simulink model "Traj_plt"  (R2023a)
settings: Solver=VariableStepAuto  StartTime=0.0  StopTime=inf  RelTol=1e-3
values from neighbouring files (symbols this model uses):
  beta = beta_i'.*task    [Compare1.m]    (also in Compare2.m; Final1.m; Final2.m; Final3.m)
undefined symbols (not defined in the file or in its folder): B_prev, Bst, Bst_prev, convertStringsToChars, dist_C, DroneMass, Earth, Gravity, h_ref, initialState, quad_pos, sinit, stack_size, task_mat, WGS84
libraries: slpidlib x66, aerolibconvert2 x11, aerolibtransform2 x11, uavalgslib x11, dspsrcs4 x1
(part 12 of 12)

== system Traj_plt/agent_9/Quad_1/Inner Loop and Plant Model/Low-FidelityModel/Position and Acceleration Control/Velocity Control1 ==
  Velocity Cmd : Inport
  QuadRotorState : Inport  Port=2
  Add1 : Sum  Inputs=+-
  Bus Selector1 : BusSelector  OutputSignals=WorldVelocity
  Data Type Conversion{,1..5} (6 alike) : DataTypeConversion  OutDataTypeStr=single  SaturateOnIntegerOverflow=off  RndMeth=Floor
  Demux1 : Demux  Outputs=3
  Mux : Mux  Inputs=3
  PID_Vx : slpidlib/PID Controller  Controller=PID  Form=Parallel  TimeDomain=Discrete-time  UseExternalTs=off  SampleTime=-1  IntegratorMethod=Forward Euler  FilterMethod=Forward Euler  ControllerParametersSource=internal  P=0.35  I=0  UseKiTs=off  D=0.1  N=10  UseFilter=on  TunerSelectOption=Transfer Function Based (PID Tuner App)  InitialConditionSource=internal  InitialConditionForIntegrator=0  InitialConditionForFilter=0  DifferentiatorICPrevScaledInput=0  ExternalReset=none  TrackingMode=off  Kt=1  LimitOutput=on  SatLimitsSource=internal  UpperSaturationLimit=1  LowerSaturationLimit=-1  LinearizeAsGain=on  AntiWindupMode=clamping  Kb=1  LimitIntegrator=off  UpperIntegratorSaturationLimit=inf  LowerIntegratorSaturationLimit=-inf  PGainOutDataTypeStr=single  PProdOutDataTypeStr=single  POutMin=[]  POutMax=[]  IGainOutDataTypeStr=single  IProdOutDataTypeStr=single  IOutMin=[]  IOutMax=[]  DGainOutDataTypeStr=single  DProdOutDataTypeStr=single  DOutMin=[]  DOutMax=[]  NGainOutDataTypeStr=single  NProdOutDataTypeStr=single  NOutMin=[]  NOutMax=[]  SumOutDataTypeStr=single  SumOutMin=[]  SumOutMax=[]  SaturationOutDataTypeStr=single  SaturationOutMin=[]  SaturationOutMax=[]  PParamMin=[]  PParamMax=[]  IParamMin=[]  IParamMax=[]  DParamMin=[]  DParamMax=[]  NParamMin=[]  NParamMax=[]  KbParamMin=[]  KbParamMax=[]  KtParamMin=[]  KtParamMax=[]  KbOutMin=[]  KbOutMax=[]  KtOutMin=[]  KtOutMax=[]  IntegratorOutMin=[]  IntegratorOutMax=[]  FilterOutMin=[]  FilterOutMax=[]  SumI1OutMin=SumI1OutMin  SumI1OutMax=SumI1OutMax  SumI2OutMin=[]  SumI2OutMax=[]  SumI3OutMin=[]  SumI3OutMax=[]  SumI4OutMin=[]  SumI4OutMax=[]  SumDOutMin=[]  SumDOutMax=[]  DifferentiatorOutMin=[]  DifferentiatorOutMax=[]  FilterDiffOutCoefMin=[]  FilterDiffOutCoefMax=[]  ReciprocalOutMin=[]  ReciprocalOutMax=[]  SumDenOutMin=[]  SumDenOutMax=[]  SumNumOutMin=[]  SumNumOutMax=[]  DivideOutMin=[]  DivideOutMax=[]  UdiffTsProdOutMin=[]  UdiffTsProdOutMax=[]  NTsProdOutMin=[]  NTsProdOutMax=[]  UintegralTsProdOutMin=[]  UintegralTsProdOutMax=[]  UngainTsProdOutMin=[]  UngainTsProdOutMax=[]  ClampingZeroOutDataTypeStr=Inherit: Inherit via back propagation  ClampingZeroOutMin=[]  ClampingZeroOutMax=[]  FilterDenConstantOutDataTypeStr=Inherit: Inherit via back propagation  FilterDenConstantOutMin=[]  FilterDenConstantOutMax=[]  PCopyOutDataTypeStr=Inherit: Inherit via back propagation  PCopyOutMin=[]  PCopyOutMax=[]  NCopyOutDataTypeStr=Inherit: Inherit via back propagation  NCopyOutMin=[]  NCopyOutMax=[]  IntegratorContinuousStateAttributes=''  IntegratorStateMustResolveToSignalObject=off  IntegratorRTWStateStorageClass=Auto  FilterContinuousStateAttributes=''  FilterStateMustResolveToSignalObject=off  FilterRTWStateStorageClass=Auto  ParallelPVariant=InternalParameters  IdealPVariant=Disabled  IVariant=InternalParameters  DVariant=InternalParameters  IntegratorVariant=Discrete  SatVariant=Enabled  AWVariant=DiscClampingParallel  PCopyVariant=Disabled  TRVariant=Disabled  FdbkBlocksVariant=Forward  IdealPFdbkVariant=Disabled  SatFdbkVariant=Disabled  DerivativeFilterVariant=ForwardEulerFilter  NVariant=InternalParameters  NCopyVariant=Disabled  FilterICVariant=InternalICsFilter  IntegratorICVariant=InternalICs  ExternalResetVariant=Disabled  TRSumVariant=Passthrough  SumFdbkVariant=Disabled  SumVariant=Sum_PID  TsampFilterVariant=InternalTs  TsampNgainVariant=Passthrough  TsampIntegralVariant=Disabled_SignalSpec  ExternalSaturationOutDataTypeStr=Inherit: Same as second input
      settings: AttributesFormatString=P: %<P>, I: %<I>, D:%<D>
  PID_Vy : slpidlib/PID Controller  Controller=PID  Form=Parallel  TimeDomain=Discrete-time  UseExternalTs=off  SampleTime=-1  IntegratorMethod=Forward Euler  FilterMethod=Forward Euler  ControllerParametersSource=internal  P=0.35  I=0  UseKiTs=off  D=0.1  N=10  UseFilter=on  TunerSelectOption=Transfer Function Based (PID Tuner App)  InitialConditionSource=internal  InitialConditionForIntegrator=0  InitialConditionForFilter=0  DifferentiatorICPrevScaledInput=0  ExternalReset=none  TrackingMode=off  Kt=1  LimitOutput=on  SatLimitsSource=internal  UpperSaturationLimit=1  LowerSaturationLimit=-1  LinearizeAsGain=on  AntiWindupMode=clamping  Kb=1  LimitIntegrator=off  UpperIntegratorSaturationLimit=inf  LowerIntegratorSaturationLimit=-inf  POutMin=[]  POutMax=[]  IOutMin=[]  IOutMax=[]  DOutMin=[]  DOutMax=[]  NOutMin=[]  NOutMax=[]  SumOutMin=[]  SumOutMax=[]  SaturationOutMin=[]  SaturationOutMax=[]  PParamMin=[]  PParamMax=[]  IParamMin=[]  IParamMax=[]  DParamMin=[]  DParamMax=[]  NParamMin=[]  NParamMax=[]  KbParamMin=[]  KbParamMax=[]  KtParamMin=[]  KtParamMax=[]  KbOutMin=[]  KbOutMax=[]  KtOutMin=[]  KtOutMax=[]  IntegratorOutMin=[]  IntegratorOutMax=[]  FilterOutMin=[]  FilterOutMax=[]  SumI1OutMin=SumI1OutMin  SumI1OutMax=SumI1OutMax  SumI2OutMin=[]  SumI2OutMax=[]  SumI3OutMin=[]  SumI3OutMax=[]  SumI4OutMin=[]  SumI4OutMax=[]  SumDOutMin=[]  SumDOutMax=[]  DifferentiatorOutMin=[]  DifferentiatorOutMax=[]  FilterDiffOutCoefMin=[]  FilterDiffOutCoefMax=[]  ReciprocalOutMin=[]  ReciprocalOutMax=[]  SumDenOutMin=[]  SumDenOutMax=[]  SumNumOutMin=[]  SumNumOutMax=[]  DivideOutMin=[]  DivideOutMax=[]  UdiffTsProdOutMin=[]  UdiffTsProdOutMax=[]  NTsProdOutMin=[]  NTsProdOutMax=[]  UintegralTsProdOutMin=[]  UintegralTsProdOutMax=[]  UngainTsProdOutMin=[]  UngainTsProdOutMax=[]  ClampingZeroOutDataTypeStr=Inherit: Inherit via back propagation  ClampingZeroOutMin=[]  ClampingZeroOutMax=[]  FilterDenConstantOutDataTypeStr=Inherit: Inherit via back propagation  FilterDenConstantOutMin=[]  FilterDenConstantOutMax=[]  PCopyOutDataTypeStr=Inherit: Inherit via back propagation  PCopyOutMin=[]  PCopyOutMax=[]  NCopyOutDataTypeStr=Inherit: Inherit via back propagation  NCopyOutMin=[]  NCopyOutMax=[]  IntegratorContinuousStateAttributes=''  IntegratorStateMustResolveToSignalObject=off  IntegratorRTWStateStorageClass=Auto  FilterContinuousStateAttributes=''  FilterStateMustResolveToSignalObject=off  FilterRTWStateStorageClass=Auto  ParallelPVariant=InternalParameters  IdealPVariant=Disabled  IVariant=InternalParameters  DVariant=InternalParameters  IntegratorVariant=Discrete  SatVariant=Enabled  AWVariant=DiscClampingParallel  PCopyVariant=Disabled  TRVariant=Disabled  FdbkBlocksVariant=Forward  IdealPFdbkVariant=Disabled  SatFdbkVariant=Disabled  DerivativeFilterVariant=ForwardEulerFilter  NVariant=InternalParameters  NCopyVariant=Disabled  FilterICVariant=InternalICsFilter  IntegratorICVariant=InternalICs  ExternalResetVariant=Disabled  TRSumVariant=Passthrough  SumFdbkVariant=Disabled  SumVariant=Sum_PID  TsampFilterVariant=InternalTs  TsampNgainVariant=Passthrough  TsampIntegralVariant=Disabled_SignalSpec  ExternalSaturationOutDataTypeStr=Inherit: Same as second input
      settings: AttributesFormatString=P: %<P>, I: %<I>, D:%<D>
  PID_Vz : slpidlib/PID Controller  Controller=PID  Form=Parallel  TimeDomain=Discrete-time  UseExternalTs=off  SampleTime=-1  IntegratorMethod=Forward Euler  FilterMethod=Forward Euler  ControllerParametersSource=internal  P=6.8  I=0  UseKiTs=off  D=2.5  N=14.495  UseFilter=on  TunerSelectOption=Transfer Function Based (PID Tuner App)  InitialConditionSource=internal  InitialConditionForIntegrator=0  InitialConditionForFilter=0  DifferentiatorICPrevScaledInput=0  ExternalReset=none  TrackingMode=off  Kt=1  LimitOutput=on  SatLimitsSource=internal  UpperSaturationLimit=2  LowerSaturationLimit=-2  LinearizeAsGain=on  AntiWindupMode=clamping  Kb=1  LimitIntegrator=off  UpperIntegratorSaturationLimit=inf  LowerIntegratorSaturationLimit=-inf  POutMin=[]  POutMax=[]  IOutMin=[]  IOutMax=[]  DOutMin=[]  DOutMax=[]  NOutMin=[]  NOutMax=[]  SumOutMin=[]  SumOutMax=[]  SaturationOutMin=[]  SaturationOutMax=[]  PParamMin=[]  PParamMax=[]  IParamMin=[]  IParamMax=[]  DParamMin=[]  DParamMax=[]  NParamMin=[]  NParamMax=[]  KbParamMin=[]  KbParamMax=[]  KtParamMin=[]  KtParamMax=[]  KbOutMin=[]  KbOutMax=[]  KtOutMin=[]  KtOutMax=[]  IntegratorOutMin=[]  IntegratorOutMax=[]  FilterOutMin=[]  FilterOutMax=[]  SumI1OutMin=SumI1OutMin  SumI1OutMax=SumI1OutMax  SumI2OutMin=[]  SumI2OutMax=[]  SumI3OutMin=[]  SumI3OutMax=[]  SumI4OutMin=[]  SumI4OutMax=[]  SumDOutMin=[]  SumDOutMax=[]  DifferentiatorOutMin=[]  DifferentiatorOutMax=[]  FilterDiffOutCoefMin=[]  FilterDiffOutCoefMax=[]  ReciprocalOutMin=[]  ReciprocalOutMax=[]  SumDenOutMin=[]  SumDenOutMax=[]  SumNumOutMin=[]  SumNumOutMax=[]  DivideOutMin=[]  DivideOutMax=[]  UdiffTsProdOutMin=[]  UdiffTsProdOutMax=[]  NTsProdOutMin=[]  NTsProdOutMax=[]  UintegralTsProdOutMin=[]  UintegralTsProdOutMax=[]  UngainTsProdOutMin=[]  UngainTsProdOutMax=[]  ClampingZeroOutDataTypeStr=Inherit: Inherit via back propagation  ClampingZeroOutMin=[]  ClampingZeroOutMax=[]  FilterDenConstantOutDataTypeStr=Inherit: Inherit via back propagation  FilterDenConstantOutMin=[]  FilterDenConstantOutMax=[]  PCopyOutDataTypeStr=Inherit: Inherit via back propagation  PCopyOutMin=[]  PCopyOutMax=[]  NCopyOutDataTypeStr=Inherit: Inherit via back propagation  NCopyOutMin=[]  NCopyOutMax=[]  IntegratorContinuousStateAttributes=''  IntegratorStateMustResolveToSignalObject=off  IntegratorRTWStateStorageClass=Auto  FilterContinuousStateAttributes=''  FilterStateMustResolveToSignalObject=off  FilterRTWStateStorageClass=Auto  ParallelPVariant=InternalParameters  IdealPVariant=Disabled  IVariant=InternalParameters  DVariant=InternalParameters  IntegratorVariant=Discrete  SatVariant=Enabled  AWVariant=DiscClampingParallel  PCopyVariant=Disabled  TRVariant=Disabled  FdbkBlocksVariant=Forward  IdealPFdbkVariant=Disabled  SatFdbkVariant=Disabled  DerivativeFilterVariant=ForwardEulerFilter  NVariant=InternalParameters  NCopyVariant=Disabled  FilterICVariant=InternalICsFilter  IntegratorICVariant=InternalICs  ExternalResetVariant=Disabled  TRSumVariant=Passthrough  SumFdbkVariant=Disabled  SumVariant=Sum_PID  TsampFilterVariant=InternalTs  TsampNgainVariant=Passthrough  TsampIntegralVariant=Disabled_SignalSpec  ExternalSaturationOutDataTypeStr=Inherit: Same as second input
      settings: AttributesFormatString=P: %<P>, I: %<I>, D:%<D>
  Accel Cmd : Outport
  wires:
  Add1/1 -> Demux1/1  "Velocity Error"
  PID_Vz/1 -> Data Type Conversion/1
  Demux1/1 -> Data Type Conversion4/1
  PID_Vy/1 -> Data Type Conversion1/1
  Velocity Cmd/1 -> Add1/1
  Demux1/3 -> Data Type Conversion5/1
  Mux/1 -> Accel Cmd/1
  PID_Vx/1 -> Data Type Conversion2/1
  Demux1/2 -> Data Type Conversion3/1
  Bus Selector1/1 -> Add1/2  "<WorldVelocity>"
  QuadRotorState/1 -> Bus Selector1/1
  Data Type Conversion/1 -> Mux/3
  Data Type Conversion1/1 -> Mux/2
  Data Type Conversion2/1 -> Mux/1
  Data Type Conversion3/1 -> PID_Vy/1
  Data Type Conversion4/1 -> PID_Vx/1
  Data Type Conversion5/1 -> PID_Vz/1

== matlab function Traj_plt/agent_11/Quad_1/Inner Loop and Plant Model/Low-FidelityModel/Assemble UAV State Bus/Generate GPS Data/Embedded MATLAB Function1 ==
  data: cog output; Vn input; Ve input
function cog = getCOG(Vn, Ve)
% This block supports an embeddable subset of the MATLAB language.
% See the help menu for details. 

cog = atan2(Ve,Vn);
if cog < 0;
    cog = cog + 2*pi;
end

== matlab function Traj_plt/MATLAB Function ==
  data: ag_no input; h output; d output; h_ref parameter; dist_C parameter
function [h,d] = fcn(ag_no, h_ref, dist_C)
h = h_ref(ag_no);
d = dist_C(ag_no);

== matlab function Traj_plt/agent_11/Quad_1/Inner Loop and Plant Model/Low-FidelityModel/Position and Acceleration Control/Attitude Control/Multirotor Acceleration Control ==
  data: acc input; roll output; pitch output; yaw input; Gravity parameter
function [roll, pitch] = accControl(acc, yaw, Gravity)

    xddot = acc(1);
    yddot = acc(2);
    zddot = acc(3);
    
    pitch = atan2((-xddot*cos(yaw)-yddot*sin(yaw)), ( -zddot + Gravity));
    roll = atan2(((-xddot*sin(yaw)+yddot*cos(yaw))*cos(pitch)), (-zddot+Gravity));
    
end

== matlab function Traj_plt/agent_11/Quad_1/Inner Loop and Plant Model/Low-FidelityModel/Position and Acceleration Control/Attitude Control/Multirotor Thrust Control ==
  data: acc input; pitch input; thrust output; roll input; DroneMass parameter; Gravity parameter
function thrust  = thrustControl(acc, pitch, roll, DroneMass, Gravity)

    zddot = acc(3);
    
    thrust = DroneMass*(-zddot+Gravity)/(cos(pitch)*cos(roll));
end

== matlab function Traj_plt/Fire_dyn ==
  data: srate output; beta input; s input
function srate = fcn(beta,s)
Fir_pts = [80,100;120,100]';
alpha = [1.2,1.5];
sinit = [2.1,1.2];
k = 0.6;
srate = k.*alpha.*sqrt(s)'-beta';
circle(Fir_pts(1,1),Fir_pts(2,1),sqrt(s(1)/pi),beta(1),s)
hold on
circle(Fir_pts(1,2),Fir_pts(2,2),sqrt(s(2)/pi),beta(2),s)
y=0;

== stateflow chart Traj_plt/Chart2 ==
  state Stat_assign
    Beta = Bst_prev*beta';
    %Bst = Bst_prev;
  state B_assign1
    Bst == task_mat(j,:,:);
  state B_assign
    Beta = Bst * beta';
  (default) -> Stat_assign
  Stat_assign -> B_assign : after(10,sec){j=1}
  B_assign -> B_assign1 : after(10,sec){j = j + 1}
  B_assign1 -> B_assign : after(1,sec)
  data: task_mat parameter; Bst_prev parameter; Bst parameter; Beta output; j output; beta parameter

== matlab function Traj_plt/agent_1/Quad_1/Inner Loop and Plant Model/Low-FidelityModel/Assemble UAV State Bus/Generate GPS Data/Embedded MATLAB Function1 ==
  data: cog output; Vn input; Ve input
function cog = getCOG(Vn, Ve)
% This block supports an embeddable subset of the MATLAB language.
% See the help menu for details. 

cog = atan2(Ve,Vn);
if cog < 0;
    cog = cog + 2*pi;
end

== matlab function Traj_plt/agent_1/Quad_1/Inner Loop and Plant Model/Low-FidelityModel/Position and Acceleration Control/Attitude Control/Multirotor Acceleration Control ==
  data: acc input; roll output; pitch output; yaw input; Gravity parameter
function [roll, pitch] = accControl(acc, yaw, Gravity)

    xddot = acc(1);
    yddot = acc(2);
    zddot = acc(3);
    
    pitch = atan2((-xddot*cos(yaw)-yddot*sin(yaw)), ( -zddot + Gravity));
    roll = atan2(((-xddot*sin(yaw)+yddot*cos(yaw))*cos(pitch)), (-zddot+Gravity));
    
end

== matlab function Traj_plt/agent_1/Quad_1/Inner Loop and Plant Model/Low-FidelityModel/Position and Acceleration Control/Attitude Control/Multirotor Thrust Control ==
  data: acc input; pitch input; thrust output; roll input; DroneMass parameter; Gravity parameter
function thrust  = thrustControl(acc, pitch, roll, DroneMass, Gravity)

    zddot = acc(3);
    
    thrust = DroneMass*(-zddot+Gravity)/(cos(pitch)*cos(roll));
end

== matlab function Traj_plt/MATLAB Function1 ==
  data: ag_no input; h output; d output; h_ref parameter; dist_C parameter
function [h,d] = fcn(ag_no, h_ref, dist_C)
h = h_ref(ag_no);
d = dist_C(ag_no);

== stateflow chart Traj_plt/agent_1/Chart2 ==
  state Stat_assign
    B = B_prev(ag_no);
  state B_assign1
    B = task_mat(j,ag_no,1);
  state B_assign
    B;
  (default) -> Stat_assign
  Stat_assign -> B_assign : after(10,sec){j=1}
  B_assign -> B_assign1 : after(10,sec){j = j + 1}
  B_assign1 -> B_assign : after(1,sec)
  data: B output; task_mat parameter; ag_no input; B_prev parameter; j output

== stateflow chart Traj_plt/agent_2/Chart1 ==
  state Fire_pt_1
    state set_1
      waypoint =[x-d,y-d,h; x+d,y-d,h;x+d,y+d,h;x-d,y+d,h];
    state set_2
      waypoint =[ x-d,y-d,h-0.1; x+d,y-d,h-0.1;x+d,y+d,h-0.1;x-d,y+d,h-0.1];
    Fire_pt_1.set_1 -> Fire_pt_1.set_2 : [meet==1]
    (default) -> Fire_pt_1.set_1
    Fire_pt_1.set_2 -> Fire_pt_1.set_1 : [meet==1]
  state Fire_pt_2
    state set_1
      waypoint =[a-d,b-d,g; a+d,b-d,g;a+d,b+d,g;a-d,b+d,g];
    state set_2
      waypoint = [ a-d,b-d,h-0.1; a+d,b-d,h-0.1;a+d,b+d,h-0.1;a-d,b+d,h-0.1];
    (default) -> Fire_pt_2.set_1
    Fire_pt_2.set_1 -> Fire_pt_2.set_2 : [meet==1]
    Fire_pt_2.set_2 -> Fire_pt_2.set_1 : [meet==1]
  (default) -> Fire_pt_1
  Fire_pt_1 -> Fire_pt_2 : [Assign==1]
  Fire_pt_2 -> Fire_pt_1 : [Assign==0]
  data: waypoint output; Assign input; a input; b input; g input; x input; h input; y input; d input; meet input

== stateflow chart Traj_plt/agent_2/Chart2 ==
  state Stat_assign
    B = B_prev(ag_no);
  state B_assign1
    B = task_mat(j,ag_no,1);
  state B_assign
    B;
  (default) -> Stat_assign
  Stat_assign -> B_assign : after(10,sec){j=1}
  B_assign -> B_assign1 : after(10,sec){j = j + 1}
  B_assign1 -> B_assign : after(1,sec)
  data: B output; task_mat parameter; ag_no input; B_prev parameter; j output

== matlab function Traj_plt/agent_2/MATLAB Function ==
  data: Assign output; B input
function Assign = fcn(B)
if (B==1)
    Assign=0;
else
    Assign=1;
end

== matlab function Traj_plt/agent_2/Quad_1/Inner Loop and Plant Model/Low-FidelityModel/Assemble UAV State Bus/Generate GPS Data/Embedded MATLAB Function1 ==
  data: cog output; Vn input; Ve input
function cog = getCOG(Vn, Ve)
% This block supports an embeddable subset of the MATLAB language.
% See the help menu for details. 

cog = atan2(Ve,Vn);
if cog < 0;
    cog = cog + 2*pi;
end

== matlab function Traj_plt/agent_2/Quad_1/Inner Loop and Plant Model/Low-FidelityModel/Position and Acceleration Control/Attitude Control/Multirotor Acceleration Control ==
  data: acc input; roll output; pitch output; yaw input; Gravity parameter
function [roll, pitch] = accControl(acc, yaw, Gravity)

    xddot = acc(1);
    yddot = acc(2);
    zddot = acc(3);
    
    pitch = atan2((-xddot*cos(yaw)-yddot*sin(yaw)), ( -zddot + Gravity));
    roll = atan2(((-xddot*sin(yaw)+yddot*cos(yaw))*cos(pitch)), (-zddot+Gravity));
    
end

== matlab function Traj_plt/agent_2/Quad_1/Inner Loop and Plant Model/Low-FidelityModel/Position and Acceleration Control/Attitude Control/Multirotor Thrust Control ==
  data: acc input; pitch input; thrust output; roll input; DroneMass parameter; Gravity parameter
function thrust  = thrustControl(acc, pitch, roll, DroneMass, Gravity)

    zddot = acc(3);
    
    thrust = DroneMass*(-zddot+Gravity)/(cos(pitch)*cos(roll));
end

== matlab function Traj_plt/MATLAB Function2 ==
  data: ag_no input; h output; d output; h_ref parameter; dist_C parameter
function [h,d] = fcn(ag_no, h_ref, dist_C)
h = h_ref(ag_no);
d = dist_C(ag_no);

== stateflow chart Traj_plt/agent_3/Chart1 ==
  state Fire_pt_1
    state set_1
      waypoint =[x-d,y-d,h; x+d,y-d,h;x+d,y+d,h;x-d,y+d,h];
    state set_2
      waypoint =[ x-d,y-d,h-0.1; x+d,y-d,h-0.1;x+d,y+d,h-0.1;x-d,y+d,h-0.1];
    Fire_pt_1.set_1 -> Fire_pt_1.set_2 : [meet==1]
    (default) -> Fire_pt_1.set_1
    Fire_pt_1.set_2 -> Fire_pt_1.set_1 : [meet==1]
  state Fire_pt_2
    state set_1
      waypoint =[a-d,b-d,g; a+d,b-d,g;a+d,b+d,g;a-d,b+d,g];
    state set_2
      waypoint = [ a-d,b-d,h-0.1; a+d,b-d,h-0.1;a+d,b+d,h-0.1;a-d,b+d,h-0.1];
    Fire_pt_2.set_1 -> Fire_pt_2.set_2 : [meet==1]
    (default) -> Fire_pt_2.set_1
    Fire_pt_2.set_2 -> Fire_pt_2.set_1 : [meet==1]
  (default) -> Fire_pt_1
  Fire_pt_1 -> Fire_pt_2 : [Assign==1]
  Fire_pt_2 -> Fire_pt_1 : [Assign==0]
  data: waypoint output; Assign input; a input; b input; g input; x input; h input; y input; d input; meet input

== stateflow chart Traj_plt/agent_3/Chart2 ==
  state Stat_assign
    B = B_prev(ag_no);
  state B_assign1
    B = task_mat(j,ag_no,1);
  state B_assign
    B;
  (default) -> Stat_assign
  Stat_assign -> B_assign : after(10,sec){j=1}
  B_assign -> B_assign1 : after(10,sec){j = j + 1}
  B_assign1 -> B_assign : after(1,sec)
  data: B output; task_mat parameter; ag_no input; B_prev parameter; j output

== matlab function Traj_plt/agent_3/MATLAB Function ==
  data: Assign output; B input
function Assign = fcn(B)
if (B==1)
    Assign=0;
else
    Assign=1;
end

== matlab function Traj_plt/agent_3/Quad_1/Inner Loop and Plant Model/Low-FidelityModel/Assemble UAV State Bus/Generate GPS Data/Embedded MATLAB Function1 ==
  data: cog output; Vn input; Ve input
function cog = getCOG(Vn, Ve)
% This block supports an embeddable subset of the MATLAB language.
% See the help menu for details. 

cog = atan2(Ve,Vn);
if cog < 0;
    cog = cog + 2*pi;
end

== matlab function Traj_plt/agent_3/Quad_1/Inner Loop and Plant Model/Low-FidelityModel/Position and Acceleration Control/Attitude Control/Multirotor Acceleration Control ==
  data: acc input; roll output; pitch output; yaw input; Gravity parameter
function [roll, pitch] = accControl(acc, yaw, Gravity)

    xddot = acc(1);
    yddot = acc(2);
    zddot = acc(3);
    
    pitch = atan2((-xddot*cos(yaw)-yddot*sin(yaw)), ( -zddot + Gravity));
    roll = atan2(((-xddot*sin(yaw)+yddot*cos(yaw))*cos(pitch)), (-zddot+Gravity));
    
end

== matlab function Traj_plt/agent_3/Quad_1/Inner Loop and Plant Model/Low-FidelityModel/Position and Acceleration Control/Attitude Control/Multirotor Thrust Control ==
  data: acc input; pitch input; thrust output; roll input; DroneMass parameter; Gravity parameter
function thrust  = thrustControl(acc, pitch, roll, DroneMass, Gravity)

    zddot = acc(3);
    
    thrust = DroneMass*(-zddot+Gravity)/(cos(pitch)*cos(roll));
end

== matlab function Traj_plt/MATLAB Function3 ==
  data: ag_no input; h output; d output; h_ref parameter; dist_C parameter
function [h,d] = fcn(ag_no, h_ref, dist_C)
h = h_ref(ag_no);
d = dist_C(ag_no);

== stateflow chart Traj_plt/agent_4/Chart1 ==
  state Fire_pt_1
    state set_1
      waypoint =[x-d,y-d,h; x+d,y-d,h;x+d,y+d,h;x-d,y+d,h];
    state set_2
      waypoint =[ x-d,y-d,h-0.1; x+d,y-d,h-0.1;x+d,y+d,h-0.1;x-d,y+d,h-0.1];
    Fire_pt_1.set_1 -> Fire_pt_1.set_2 : [meet==1]
    (default) -> Fire_pt_1.set_1
    Fire_pt_1.set_2 -> Fire_pt_1.set_1 : [meet==1]
  state Fire_pt_2
    state set_1
      waypoint =[a-d,b-d,g; a+d,b-d,g;a+d,b+d,g;a-d,b+d,g];
    state set_2
      waypoint = [ a-d,b-d,h-0.1; a+d,b-d,h-0.1;a+d,b+d,h-0.1;a-d,b+d,h-0.1];
    Fire_pt_2.set_1 -> Fire_pt_2.set_2 : [meet==1]
    (default) -> Fire_pt_2.set_1
    Fire_pt_2.set_2 -> Fire_pt_2.set_1 : [meet==1]
  (default) -> Fire_pt_1
  Fire_pt_1 -> Fire_pt_2 : [Assign==1]
  Fire_pt_2 -> Fire_pt_1 : [Assign==0]
  data: waypoint output; Assign input; a input; b input; g input; x input; h input; y input; d input; meet input

== stateflow chart Traj_plt/agent_4/Chart2 ==
  state Stat_assign
    B = B_prev(ag_no);
  state B_assign1
    B = task_mat(j,ag_no,1);
  state B_assign
    B;
  (default) -> Stat_assign
  Stat_assign -> B_assign : after(10,sec){j=1}
  B_assign -> B_assign1 : after(10,sec){j = j + 1}
  B_assign1 -> B_assign : after(1,sec)
  data: B output; task_mat parameter; ag_no input; B_prev parameter; j output

== matlab function Traj_plt/agent_4/MATLAB Function ==
  data: Assign output; B input
function Assign = fcn(B)
if (B==1)
    Assign=0;
else
    Assign=1;
end

== matlab function Traj_plt/agent_4/Quad_1/Inner Loop and Plant Model/Low-FidelityModel/Assemble UAV State Bus/Generate GPS Data/Embedded MATLAB Function1 ==
  data: cog output; Vn input; Ve input
function cog = getCOG(Vn, Ve)
% This block supports an embeddable subset of the MATLAB language.
% See the help menu for details. 

cog = atan2(Ve,Vn);
if cog < 0;
    cog = cog + 2*pi;
end

== matlab function Traj_plt/agent_4/Quad_1/Inner Loop and Plant Model/Low-FidelityModel/Position and Acceleration Control/Attitude Control/Multirotor Acceleration Control ==
  data: acc input; roll output; pitch output; yaw input; Gravity parameter
function [roll, pitch] = accControl(acc, yaw, Gravity)

    xddot = acc(1);
    yddot = acc(2);
    zddot = acc(3);
    
    pitch = atan2((-xddot*cos(yaw)-yddot*sin(yaw)), ( -zddot + Gravity));
    roll = atan2(((-xddot*sin(yaw)+yddot*cos(yaw))*cos(pitch)), (-zddot+Gravity));
    
end

== matlab function Traj_plt/agent_4/Quad_1/Inner Loop and Plant Model/Low-FidelityModel/Position and Acceleration Control/Attitude Control/Multirotor Thrust Control ==
  data: acc input; pitch input; thrust output; roll input; DroneMass parameter; Gravity parameter
function thrust  = thrustControl(acc, pitch, roll, DroneMass, Gravity)

    zddot = acc(3);
    
    thrust = DroneMass*(-zddot+Gravity)/(cos(pitch)*cos(roll));
end

== matlab function Traj_plt/MATLAB Function4 ==
  data: ag_no input; h output; d output; h_ref parameter; dist_C parameter
function [h,d] = fcn(ag_no, h_ref, dist_C)
h = h_ref(ag_no);
d = dist_C(ag_no);

== stateflow chart Traj_plt/agent_5/Chart1 ==
  state Fire_pt_1
    state set_1
      waypoint =[x-d,y-d,h; x+d,y-d,h;x+d,y+d,h;x-d,y+d,h];
    state set_2
      waypoint =[ x-d,y-d,h-0.1; x+d,y-d,h-0.1;x+d,y+d,h-0.1;x-d,y+d,h-0.1];
    Fire_pt_1.set_1 -> Fire_pt_1.set_2 : [meet==1]
    (default) -> Fire_pt_1.set_1
    Fire_pt_1.set_2 -> Fire_pt_1.set_1 : [meet==1]
  state Fire_pt_2
    state set_1
      waypoint =[a-d,b-d,g; a+d,b-d,g;a+d,b+d,g;a-d,b+d,g];
    state set_2
      waypoint = [ a-d,b-d,h-0.1; a+d,b-d,h-0.1;a+d,b+d,h-0.1;a-d,b+d,h-0.1];
    Fire_pt_2.set_1 -> Fire_pt_2.set_2 : [meet==1]
    (default) -> Fire_pt_2.set_1
    Fire_pt_2.set_2 -> Fire_pt_2.set_1 : [meet==1]
  (default) -> Fire_pt_1
  Fire_pt_1 -> Fire_pt_2 : [Assign==1]
  Fire_pt_2 -> Fire_pt_1 : [Assign==0]
  data: waypoint output; Assign input; a input; b input; g input; x input; h input; y input; d input; meet input

== stateflow chart Traj_plt/agent_5/Chart2 ==
  state Stat_assign
    B = B_prev(ag_no);
  state B_assign1
    B = task_mat(j,ag_no,1);
  state B_assign
    B;
  (default) -> Stat_assign
  Stat_assign -> B_assign : after(10,sec){j=1}
  B_assign -> B_assign1 : after(10,sec){j = j + 1}
  B_assign1 -> B_assign : after(1,sec)
  data: B output; task_mat parameter; ag_no input; B_prev parameter; j output

== matlab function Traj_plt/agent_5/MATLAB Function ==
  data: Assign output; B input
function Assign = fcn(B)
if (B==1)
    Assign=0;
else
    Assign=1;
end

== matlab function Traj_plt/agent_5/Quad_1/Inner Loop and Plant Model/Low-FidelityModel/Assemble UAV State Bus/Generate GPS Data/Embedded MATLAB Function1 ==
  data: cog output; Vn input; Ve input
function cog = getCOG(Vn, Ve)
% This block supports an embeddable subset of the MATLAB language.
% See the help menu for details. 

cog = atan2(Ve,Vn);
if cog < 0;
    cog = cog + 2*pi;
end

== matlab function Traj_plt/agent_5/Quad_1/Inner Loop and Plant Model/Low-FidelityModel/Position and Acceleration Control/Attitude Control/Multirotor Acceleration Control ==
  data: acc input; roll output; pitch output; yaw input; Gravity parameter
function [roll, pitch] = accControl(acc, yaw, Gravity)

    xddot = acc(1);
    yddot = acc(2);
    zddot = acc(3);
    
    pitch = atan2((-xddot*cos(yaw)-yddot*sin(yaw)), ( -zddot + Gravity));
    roll = atan2(((-xddot*sin(yaw)+yddot*cos(yaw))*cos(pitch)), (-zddot+Gravity));
    
end

== matlab function Traj_plt/agent_5/Quad_1/Inner Loop and Plant Model/Low-FidelityModel/Position and Acceleration Control/Attitude Control/Multirotor Thrust Control ==
  data: acc input; pitch input; thrust output; roll input; DroneMass parameter; Gravity parameter
function thrust  = thrustControl(acc, pitch, roll, DroneMass, Gravity)

    zddot = acc(3);
    
    thrust = DroneMass*(-zddot+Gravity)/(cos(pitch)*cos(roll));
end

== matlab function Traj_plt/MATLAB Function5 ==
  data: ag_no input; h output; d output; h_ref parameter; dist_C parameter
function [h,d] = fcn(ag_no, h_ref, dist_C)
h = h_ref(ag_no);
d = dist_C(ag_no);

== matlab function Traj_plt/MATLAB Function6 ==
  data: ag_no input; h output; d output; h_ref parameter; dist_C parameter
function [h,d] = fcn(ag_no, h_ref, dist_C)
h = h_ref(ag_no);
d = dist_C(ag_no);

== matlab function Traj_plt/MATLAB Function7 ==
  data: ag_no input; h output; d output; h_ref parameter; dist_C parameter
function [h,d] = fcn(ag_no, h_ref, dist_C)
h = h_ref(ag_no);
d = dist_C(ag_no);

== matlab function Traj_plt/MATLAB Function8 ==
  data: ag_no input; h output; d output; h_ref parameter; dist_C parameter
function [h,d] = fcn(ag_no, h_ref, dist_C)
h = h_ref(ag_no);
d = dist_C(ag_no);

== matlab function Traj_plt/MATLAB Function9 ==
  data: ag_no input; h output; d output; h_ref parameter; dist_C parameter
function [h,d] = fcn(ag_no, h_ref, dist_C)
h = h_ref(ag_no);
d = dist_C(ag_no);

== stateflow chart Traj_plt/agent_10/Chart1 ==
  state Fire_pt_1
    state set_1
      waypoint =[x-d,y-d,h; x+d,y-d,h;x+d,y+d,h;x-d,y+d,h];
    state set_2
      waypoint =[ x-d,y-d,h-0.1; x+d,y-d,h-0.1;x+d,y+d,h-0.1;x-d,y+d,h-0.1];
    Fire_pt_1.set_1 -> Fire_pt_1.set_2 : [meet==1]
    (default) -> Fire_pt_1.set_1
    Fire_pt_1.set_2 -> Fire_pt_1.set_1 : [meet==1]
  state Fire_pt_2
    state set_1
      waypoint =[a-d,b-d,g; a+d,b-d,g;a+d,b+d,g;a-d,b+d,g];
    state set_2
      waypoint = [ a-d,b-d,h-0.1; a+d,b-d,h-0.1;a+d,b+d,h-0.1;a-d,b+d,h-0.1];
    Fire_pt_2.set_1 -> Fire_pt_2.set_2 : [meet==1]
    (default) -> Fire_pt_2.set_1
    Fire_pt_2.set_2 -> Fire_pt_2.set_1 : [meet==1]
  (default) -> Fire_pt_1
  Fire_pt_1 -> Fire_pt_2 : [Assign==1]
  Fire_pt_2 -> Fire_pt_1 : [Assign==0]
  data: waypoint output; Assign input; a input; b input; g input; x input; h input; y input; d input; meet input

== stateflow chart Traj_plt/agent_10/Chart2 ==
  state Stat_assign
    B = B_prev(ag_no);
  state B_assign1
    B = task_mat(j,ag_no,1);
  state B_assign
    B;
  (default) -> Stat_assign
  Stat_assign -> B_assign : after(10,sec){j=1}
  B_assign -> B_assign1 : after(10,sec){j = j + 1}
  B_assign1 -> B_assign : after(1,sec)
  data: B output; task_mat parameter; ag_no input; B_prev parameter; j output

== matlab function Traj_plt/agent_10/MATLAB Function ==
  data: Assign output; B input
function Assign = fcn(B)
if (B==1)
    Assign=0;
else
    Assign=1;
end

== matlab function Traj_plt/agent_10/Quad_1/Inner Loop and Plant Model/Low-FidelityModel/Assemble UAV State Bus/Generate GPS Data/Embedded MATLAB Function1 ==
  data: cog output; Vn input; Ve input
function cog = getCOG(Vn, Ve)
% This block supports an embeddable subset of the MATLAB language.
% See the help menu for details. 

cog = atan2(Ve,Vn);
if cog < 0;
    cog = cog + 2*pi;
end

== matlab function Traj_plt/agent_10/Quad_1/Inner Loop and Plant Model/Low-FidelityModel/Position and Acceleration Control/Attitude Control/Multirotor Acceleration Control ==
  data: acc input; roll output; pitch output; yaw input; Gravity parameter
function [roll, pitch] = accControl(acc, yaw, Gravity)

    xddot = acc(1);
    yddot = acc(2);
    zddot = acc(3);
    
    pitch = atan2((-xddot*cos(yaw)-yddot*sin(yaw)), ( -zddot + Gravity));
    roll = atan2(((-xddot*sin(yaw)+yddot*cos(yaw))*cos(pitch)), (-zddot+Gravity));
    
end

== matlab function Traj_plt/agent_10/Quad_1/Inner Loop and Plant Model/Low-FidelityModel/Position and Acceleration Control/Attitude Control/Multirotor Thrust Control ==
  data: acc input; pitch input; thrust output; roll input; DroneMass parameter; Gravity parameter
function thrust  = thrustControl(acc, pitch, roll, DroneMass, Gravity)

    zddot = acc(3);
    
    thrust = DroneMass*(-zddot+Gravity)/(cos(pitch)*cos(roll));
end

== stateflow chart Traj_plt/agent_6/Chart1 ==
  state Fire_pt_1
    state set_1
      waypoint =[x-d,y-d,h; x+d,y-d,h;x+d,y+d,h;x-d,y+d,h];
    state set_2
      waypoint =[ x-d,y-d,h-0.1; x+d,y-d,h-0.1;x+d,y+d,h-0.1;x-d,y+d,h-0.1];
    Fire_pt_1.set_1 -> Fire_pt_1.set_2 : [meet==1]
    (default) -> Fire_pt_1.set_1
    Fire_pt_1.set_2 -> Fire_pt_1.set_1 : [meet==1]
  state Fire_pt_2
    state set_1
      waypoint =[a-d,b-d,g; a+d,b-d,g;a+d,b+d,g;a-d,b+d,g];
    state set_2
      waypoint = [ a-d,b-d,h-0.1; a+d,b-d,h-0.1;a+d,b+d,h-0.1;a-d,b+d,h-0.1];
    (default) -> Fire_pt_2.set_1
    Fire_pt_2.set_1 -> Fire_pt_2.set_2 : [meet==1]
    Fire_pt_2.set_2 -> Fire_pt_2.set_1 : [meet==1]
  (default) -> Fire_pt_1
  Fire_pt_1 -> Fire_pt_2 : [Assign==1]
  Fire_pt_2 -> Fire_pt_1 : [Assign==0]
  data: waypoint output; Assign input; a input; b input; g input; x input; h input; y input; d input; meet input

== stateflow chart Traj_plt/agent_6/Chart2 ==
  state Stat_assign
    B = B_prev(ag_no);
  state B_assign1
    B = task_mat(j,ag_no,1);
  state B_assign
    B;
  (default) -> Stat_assign
  Stat_assign -> B_assign : after(10,sec){j=1}
  B_assign -> B_assign1 : after(10,sec){j = j + 1}
  B_assign1 -> B_assign : after(1,sec)
  data: B output; task_mat parameter; ag_no input; B_prev parameter; j output

== stateflow chart Traj_plt/agent_1/Chart1 ==
  state Fire_pt_1
    state set_1
      waypoint =[x-d,y-d,h; x+d,y-d,h;x+d,y+d,h;x-d,y+d,h];
    state set_2
      waypoint =[ x-d,y-d,h-0.1; x+d,y-d,h-0.1;x+d,y+d,h-0.1;x-d,y+d,h-0.1];
    Fire_pt_1.set_1 -> Fire_pt_1.set_2 : [meet==1]
    (default) -> Fire_pt_1.set_1
    Fire_pt_1.set_2 -> Fire_pt_1.set_1 : [meet==1]
  state Fire_pt_2
    state set_1
      waypoint =[a-d,b-d,g; a+d,b-d,g;a+d,b+d,g;a-d,b+d,g];
    state set_2
      waypoint = [ a-d,b-d,h-0.1; a+d,b-d,h-0.1;a+d,b+d,h-0.1;a-d,b+d,h-0.1];
    (default) -> Fire_pt_2.set_1
    Fire_pt_2.set_1 -> Fire_pt_2.set_2 : [meet==1]
    Fire_pt_2.set_2 -> Fire_pt_2.set_1 : [meet==1]
  (default) -> Fire_pt_1
  Fire_pt_1 -> Fire_pt_2 : [Assign==1]
  Fire_pt_2 -> Fire_pt_1 : [Assign==0]
  data: waypoint output; Assign input; a input; b input; g input; x input; h input; y input; d input; meet input

== matlab function Traj_plt/agent_6/MATLAB Function ==
  data: Assign output; B input
function Assign = fcn(B)
if (B==1)
    Assign=0;
else
    Assign=1;
end

== matlab function Traj_plt/agent_6/Quad_1/Inner Loop and Plant Model/Low-FidelityModel/Assemble UAV State Bus/Generate GPS Data/Embedded MATLAB Function1 ==
  data: cog output; Vn input; Ve input
function cog = getCOG(Vn, Ve)
% This block supports an embeddable subset of the MATLAB language.
% See the help menu for details. 

cog = atan2(Ve,Vn);
if cog < 0;
    cog = cog + 2*pi;
end

== matlab function Traj_plt/agent_6/Quad_1/Inner Loop and Plant Model/Low-FidelityModel/Position and Acceleration Control/Attitude Control/Multirotor Acceleration Control ==
  data: acc input; roll output; pitch output; yaw input; Gravity parameter
function [roll, pitch] = accControl(acc, yaw, Gravity)

    xddot = acc(1);
    yddot = acc(2);
    zddot = acc(3);
    
    pitch = atan2((-xddot*cos(yaw)-yddot*sin(yaw)), ( -zddot + Gravity));
    roll = atan2(((-xddot*sin(yaw)+yddot*cos(yaw))*cos(pitch)), (-zddot+Gravity));
    
end

== matlab function Traj_plt/agent_6/Quad_1/Inner Loop and Plant Model/Low-FidelityModel/Position and Acceleration Control/Attitude Control/Multirotor Thrust Control ==
  data: acc input; pitch input; thrust output; roll input; DroneMass parameter; Gravity parameter
function thrust  = thrustControl(acc, pitch, roll, DroneMass, Gravity)

    zddot = acc(3);
    
    thrust = DroneMass*(-zddot+Gravity)/(cos(pitch)*cos(roll));
end

== stateflow chart Traj_plt/agent_7/Chart1 ==
  state Fire_pt_1
    state set_1
      waypoint =[x-d,y-d,h; x+d,y-d,h;x+d,y+d,h;x-d,y+d,h];
    state set_2
      waypoint =[ x-d,y-d,h-0.1; x+d,y-d,h-0.1;x+d,y+d,h-0.1;x-d,y+d,h-0.1];
    Fire_pt_1.set_1 -> Fire_pt_1.set_2 : [meet==1]
    (default) -> Fire_pt_1.set_1
    Fire_pt_1.set_2 -> Fire_pt_1.set_1 : [meet==1]
  state Fire_pt_2
    state set_1
      waypoint =[a-d,b-d,g; a+d,b-d,g;a+d,b+d,g;a-d,b+d,g];
    state set_2
      waypoint = [ a-d,b-d,h-0.1; a+d,b-d,h-0.1;a+d,b+d,h-0.1;a-d,b+d,h-0.1];
    Fire_pt_2.set_1 -> Fire_pt_2.set_2 : [meet==1]
    (default) -> Fire_pt_2.set_1
    Fire_pt_2.set_2 -> Fire_pt_2.set_1 : [meet==1]
  (default) -> Fire_pt_1
  Fire_pt_1 -> Fire_pt_2 : [Assign==1]
  Fire_pt_2 -> Fire_pt_1 : [Assign==0]
  data: waypoint output; Assign input; a input; b input; g input; x input; h input; y input; d input; meet input

== stateflow chart Traj_plt/agent_7/Chart2 ==
  state Stat_assign
    B = B_prev(ag_no);
  state B_assign1
    B = task_mat(j,ag_no,1);
  state B_assign
    B;
  (default) -> Stat_assign
  Stat_assign -> B_assign : after(10,sec){j=1}
  B_assign -> B_assign1 : after(10,sec){j = j + 1}
  B_assign1 -> B_assign : after(1,sec)
  data: B output; task_mat parameter; ag_no input; B_prev parameter; j output

== matlab function Traj_plt/agent_7/MATLAB Function ==
  data: Assign output; B input
function Assign = fcn(B)
if (B==1)
    Assign=0;
else
    Assign=1;
end

== matlab function Traj_plt/agent_7/Quad_1/Inner Loop and Plant Model/Low-FidelityModel/Assemble UAV State Bus/Generate GPS Data/Embedded MATLAB Function1 ==
  data: cog output; Vn input; Ve input
function cog = getCOG(Vn, Ve)
% This block supports an embeddable subset of the MATLAB language.
% See the help menu for details. 

cog = atan2(Ve,Vn);
if cog < 0;
    cog = cog + 2*pi;
end

== matlab function Traj_plt/agent_7/Quad_1/Inner Loop and Plant Model/Low-FidelityModel/Position and Acceleration Control/Attitude Control/Multirotor Acceleration Control ==
  data: acc input; roll output; pitch output; yaw input; Gravity parameter
function [roll, pitch] = accControl(acc, yaw, Gravity)

    xddot = acc(1);
    yddot = acc(2);
    zddot = acc(3);
    
    pitch = atan2((-xddot*cos(yaw)-yddot*sin(yaw)), ( -zddot + Gravity));
    roll = atan2(((-xddot*sin(yaw)+yddot*cos(yaw))*cos(pitch)), (-zddot+Gravity));
    
end

== matlab function Traj_plt/agent_7/Quad_1/Inner Loop and Plant Model/Low-FidelityModel/Position and Acceleration Control/Attitude Control/Multirotor Thrust Control ==
  data: acc input; pitch input; thrust output; roll input; DroneMass parameter; Gravity parameter
function thrust  = thrustControl(acc, pitch, roll, DroneMass, Gravity)

    zddot = acc(3);
    
    thrust = DroneMass*(-zddot+Gravity)/(cos(pitch)*cos(roll));
end

== stateflow chart Traj_plt/agent_8/Chart1 ==
  state Fire_pt_1
    state set_1
      waypoint =[x-d,y-d,h; x+d,y-d,h;x+d,y+d,h;x-d,y+d,h];
    state set_2
      waypoint =[ x-d,y-d,h-0.1; x+d,y-d,h-0.1;x+d,y+d,h-0.1;x-d,y+d,h-0.1];
    Fire_pt_1.set_1 -> Fire_pt_1.set_2 : [meet==1]
    (default) -> Fire_pt_1.set_1
    Fire_pt_1.set_2 -> Fire_pt_1.set_1 : [meet==1]
  state Fire_pt_2
    state set_1
      waypoint =[a-d,b-d,g; a+d,b-d,g;a+d,b+d,g;a-d,b+d,g];
    state set_2
      waypoint = [ a-d,b-d,h-0.1; a+d,b-d,h-0.1;a+d,b+d,h-0.1;a-d,b+d,h-0.1];
    (default) -> Fire_pt_2.set_1
    Fire_pt_2.set_1 -> Fire_pt_2.set_2 : [meet==1]
    Fire_pt_2.set_2 -> Fire_pt_2.set_1 : [meet==1]
  (default) -> Fire_pt_1
  Fire_pt_1 -> Fire_pt_2 : [Assign==1]
  Fire_pt_2 -> Fire_pt_1 : [Assign==0]
  data: waypoint output; Assign input; a input; b input; g input; x input; h input; y input; d input; meet input

== stateflow chart Traj_plt/agent_8/Chart2 ==
  state Stat_assign
    B = B_prev(ag_no);
  state B_assign1
    B = task_mat(j,ag_no,1);
  state B_assign
    B;
  (default) -> Stat_assign
  Stat_assign -> B_assign : after(10,sec){j=1}
  B_assign -> B_assign1 : after(10,sec){j = j + 1}
  B_assign1 -> B_assign : after(1,sec)
  data: B output; task_mat parameter; ag_no input; B_prev parameter; j output

== matlab function Traj_plt/agent_8/MATLAB Function ==
  data: Assign output; B input
function Assign = fcn(B)
if (B==1)
    Assign=0;
else
    Assign=1;
end

== matlab function Traj_plt/agent_8/Quad_1/Inner Loop and Plant Model/Low-FidelityModel/Assemble UAV State Bus/Generate GPS Data/Embedded MATLAB Function1 ==
  data: cog output; Vn input; Ve input
function cog = getCOG(Vn, Ve)
% This block supports an embeddable subset of the MATLAB language.
% See the help menu for details. 

cog = atan2(Ve,Vn);
if cog < 0;
    cog = cog + 2*pi;
end

== matlab function Traj_plt/agent_8/Quad_1/Inner Loop and Plant Model/Low-FidelityModel/Position and Acceleration Control/Attitude Control/Multirotor Acceleration Control ==
  data: acc input; roll output; pitch output; yaw input; Gravity parameter
function [roll, pitch] = accControl(acc, yaw, Gravity)

    xddot = acc(1);
    yddot = acc(2);
    zddot = acc(3);
    
    pitch = atan2((-xddot*cos(yaw)-yddot*sin(yaw)), ( -zddot + Gravity));
    roll = atan2(((-xddot*sin(yaw)+yddot*cos(yaw))*cos(pitch)), (-zddot+Gravity));
    
end

== matlab function Traj_plt/agent_8/Quad_1/Inner Loop and Plant Model/Low-FidelityModel/Position and Acceleration Control/Attitude Control/Multirotor Thrust Control ==
  data: acc input; pitch input; thrust output; roll input; DroneMass parameter; Gravity parameter
function thrust  = thrustControl(acc, pitch, roll, DroneMass, Gravity)

    zddot = acc(3);
    
    thrust = DroneMass*(-zddot+Gravity)/(cos(pitch)*cos(roll));
end

== stateflow chart Traj_plt/agent_9/Chart1 ==
  state Fire_pt_1
    state set_1
      waypoint =[x-d,y-d,h; x+d,y-d,h;x+d,y+d,h;x-d,y+d,h];
    state set_2
      waypoint =[ x-d,y-d,h-0.1; x+d,y-d,h-0.1;x+d,y+d,h-0.1;x-d,y+d,h-0.1];
    Fire_pt_1.set_1 -> Fire_pt_1.set_2 : [meet==1]
    (default) -> Fire_pt_1.set_1
    Fire_pt_1.set_2 -> Fire_pt_1.set_1 : [meet==1]
  state Fire_pt_2
    state set_1
      waypoint =[a-d,b-d,g; a+d,b-d,g;a+d,b+d,g;a-d,b+d,g];
    state set_2
      waypoint = [ a-d,b-d,h-0.1; a+d,b-d,h-0.1;a+d,b+d,h-0.1;a-d,b+d,h-0.1];
    Fire_pt_2.set_1 -> Fire_pt_2.set_2 : [meet==1]
    (default) -> Fire_pt_2.set_1
    Fire_pt_2.set_2 -> Fire_pt_2.set_1 : [meet==1]
  (default) -> Fire_pt_1
  Fire_pt_1 -> Fire_pt_2 : [Assign==1]
  Fire_pt_2 -> Fire_pt_1 : [Assign==0]
  data: waypoint output; Assign input; a input; b input; g input; x input; h input; y input; d input; meet input

== stateflow chart Traj_plt/agent_9/Chart2 ==
  state Stat_assign
    B = B_prev(ag_no);
  state B_assign1
    B = task_mat(j,ag_no,1);
  state B_assign
    B;
  (default) -> Stat_assign
  Stat_assign -> B_assign : after(10,sec){j=1}
  B_assign -> B_assign1 : after(10,sec){j = j + 1}
  B_assign1 -> B_assign : after(1,sec)
  data: B output; task_mat parameter; ag_no input; B_prev parameter; j output

== matlab function Traj_plt/agent_9/MATLAB Function ==
  data: Assign output; B input
function Assign = fcn(B)
if (B==1)
    Assign=0;
else
    Assign=1;
end

== matlab function Traj_plt/agent_9/Quad_1/Inner Loop and Plant Model/Low-FidelityModel/Assemble UAV State Bus/Generate GPS Data/Embedded MATLAB Function1 ==
  data: cog output; Vn input; Ve input
function cog = getCOG(Vn, Ve)
% This block supports an embeddable subset of the MATLAB language.
% See the help menu for details. 

cog = atan2(Ve,Vn);
if cog < 0;
    cog = cog + 2*pi;
end

== matlab function Traj_plt/agent_9/Quad_1/Inner Loop and Plant Model/Low-FidelityModel/Position and Acceleration Control/Attitude Control/Multirotor Acceleration Control ==
  data: acc input; roll output; pitch output; yaw input; Gravity parameter
function [roll, pitch] = accControl(acc, yaw, Gravity)

    xddot = acc(1);
    yddot = acc(2);
    zddot = acc(3);
    
    pitch = atan2((-xddot*cos(yaw)-yddot*sin(yaw)), ( -zddot + Gravity));
    roll = atan2(((-xddot*sin(yaw)+yddot*cos(yaw))*cos(pitch)), (-zddot+Gravity));
    
end

== matlab function Traj_plt/agent_9/Quad_1/Inner Loop and Plant Model/Low-FidelityModel/Position and Acceleration Control/Attitude Control/Multirotor Thrust Control ==
  data: acc input; pitch input; thrust output; roll input; DroneMass parameter; Gravity parameter
function thrust  = thrustControl(acc, pitch, roll, DroneMass, Gravity)

    zddot = acc(3);
    
    thrust = DroneMass*(-zddot+Gravity)/(cos(pitch)*cos(roll));
end

== matlab function Traj_plt/MATLAB Function10 ==
  data: pose1 input; y output; pose2 input; pose3 input; pose4 input; pose5 input; pose6 input; pose7 input; pose8 input; pose9 input; pose10 input; quad_pos parameter
function y = fcn(pose1,pose2,pose3,pose4,pose5,pose6,pose7,pose8,pose9,pose10, quad_pos)
% set(0,'DefaultLineLineWidth', 2)
% set(0,'DefaultaxesLineWidth', 2)
% set(0,'DefaultaxesFontSize', 14)
% set(0,'DefaultTextFontSize', 14)
% set(0,'DefaultaxesFontName', 'arial');
coder.extrinsic('plot3');
plot3(pose1(1),pose1(2),pose1(3),'g+')
hold on
plot3(pose2(1),pose2(2),pose2(3),'b+')
plot3(pose3(1),pose3(2),pose3(3),'m+')
plot3(pose4(1),pose4(2),pose4(3),'c+')
plot3(pose5(1),pose5(2),pose5(3),'y+')
plot3(pose6(1),pose6(2),pose6(3),'MarkerFace',[0 0.9 0.8])
plot3(pose7(1),pose7(2),pose7(3),'MarkerFace',[0 0.7 0.7])
plot3(pose8(1),pose8(2),pose8(3),'MarkerFace',[0.6350 0.0780 0.1840])
plot3(pose9(1),pose9(2),pose9(3),'MarkerFace',[0.4660 0.6740 0.1880])
plot3(pose10(1),pose10(2),pose10(3),'MarkerFace',[0.8500 0.3250 0.0980])

plot3(quad_pos(1,2),quad_pos(2,2),quad_pos(3,2),'k*')
plot3(quad_pos(1,3),quad_pos(2,3),quad_pos(3,3),'k*')
plot3(quad_pos(1,4),quad_pos(2,4),quad_pos(3,4),'k*')
plot3(quad_pos(1,5),quad_pos(2,5),quad_pos(3,5),'k*')
plot3(quad_pos(1,6),quad_pos(2,6),quad_pos(3,6),'k*')
plot3(quad_pos(1,7),quad_pos(2,7),quad_pos(3,7),'k*')
plot3(quad_pos(1,8),quad_pos(2,8),quad_pos(3,8),'k*')
plot3(quad_pos(1,9),quad_pos(2,9),quad_pos(3,9),'k*')
plot3(quad_pos(1,10),quad_pos(2,10),quad_pos(3,10),'k*')

plot(170,150,'r*');
plot(120,100,'r*');
y=1;

== matlab function Traj_plt/agent_1/MATLAB Function ==
  data: Assign output; B input
function Assign = fcn(B)
if (B==1)
    Assign=0;
else
    Assign=1;
end

== stateflow chart Traj_plt/agent_11/Chart1 ==
  state Fire_pt_1
    state set_1
      waypoint =[x-d,y-d,h; x+d,y-d,h;x+d,y+d,h;x-d,y+d,h];
    state set_2
      waypoint =[ x-d,y-d,h-0.1; x+d,y-d,h-0.1;x+d,y+d,h-0.1;x-d,y+d,h-0.1];;
    Fire_pt_1.set_1 -> Fire_pt_1.set_2 : [meet==1]
    (default) -> Fire_pt_1.set_1
    Fire_pt_1.set_2 -> Fire_pt_1.set_1 : [meet==1]
  state Fire_pt_2
    state set_1
      waypoint =[a-d,b-d,g; a+d,b-d,g;a+d,b+d,g;a-d,b+d,g];
    state set_2
      waypoint = [ a-d,b-d,h-0.1; a+d,b-d,h-0.1;a+d,b+d,h-0.1;a-d,b+d,h-0.1];
    (default) -> Fire_pt_2.set_1
    Fire_pt_2.set_1 -> Fire_pt_2.set_2 : [meet==1]
    Fire_pt_2.set_2 -> Fire_pt_2.set_1 : [meet==1]
  (default) -> Fire_pt_1
  Fire_pt_1 -> Fire_pt_2 : [Assign==1]
  Fire_pt_2 -> Fire_pt_1 : [Assign==0]
  data: waypoint output; Assign input; a input; b input; g input; x input; h input; y input; d input; meet input

== stateflow chart Traj_plt/agent_11/Chart2 ==
  state Stat_assign
    B = B_prev(ag_no);
  state B_assign1
    B = task_mat(j,ag_no,1);
  state B_assign
    B;
  (default) -> Stat_assign
  Stat_assign -> B_assign : after(10,sec){j=1}
  B_assign -> B_assign1 : after(10,sec){j = j + 1}
  B_assign1 -> B_assign : after(1,sec)
  data: B output; task_mat parameter; ag_no input; B_prev parameter; j output

== matlab function Traj_plt/agent_11/MATLAB Function ==
  data: Assign output; B input
function Assign = fcn(B)
if (B==1)
    Assign=0;
else
    Assign=1;
end
